simulink model "MRAC_111_8_5"  (Simulink 8.9)
settings: Solver=ode45  StartTime=0.0  StopTime=40.0  RelTol=1e-3  AbsTol=1e-6
values from neighbouring files (symbols this model uses):
  af = af2    [simu_gradiente.m]
  As = 0    [parameters.m]
  DC = 1    [parameters.m]
  gamma = gamma2    [simu_gradiente.m]
  m_type = 2    [simu_gradiente.m]
  st = 0.05    [simu_gradiente.m]
  theta0 = 0    [parameters.m]
  ws = 2    [parameters.m]
libraries: cstblocks x2
settings Model: Creator=Ramon  LastModifiedBy=renan
settings DataIOCC: LimitDataPoints=off  SaveOutput=off  SaveTime=off
settings OptimizationCC: BlockReduction=off  BooleanDataType=off  ExpressionDepthLimit=2147483647  InitFltsAndDblsToZero=on
settings DebuggingCC: SaveWithParameterizedLinksMsg=none  SignalResolutionControl=TryResolveAllWithWarning  MultiTaskDSMMsg=warning  MultiTaskCondExecSysMsg=none
settings HardwareCC: TargetUnknown=on
settings RTWCC: TemplateMakefile=grt_vc.tmf

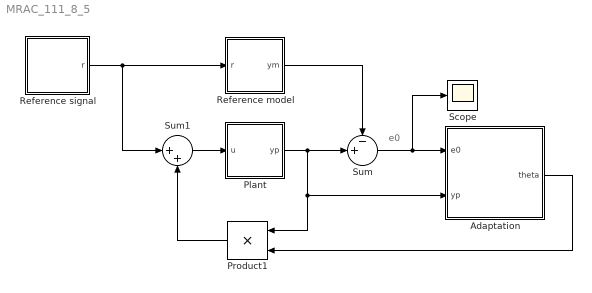
== system MRAC_111_8_5 ==
  note: e0
  Adaptation : Subsystem
  Plant : Subsystem
  Product1 : Product  SaturateOnIntegerOverflow=on  RndMeth=Zero  InputSameDT=on  OutDataTypeStr=Inherit: Same as first input
  Reference model : Subsystem
  Reference signal : Subsystem
  Scope : Scope
  Sum : Sum  Inputs=-+|  SaturateOnIntegerOverflow=on  InputSameDT=on  OutDataTypeStr=Inherit: Same as first input
  Sum1 : Sum  Inputs=|++  SaturateOnIntegerOverflow=on  InputSameDT=on  OutDataTypeStr=Inherit: Same as first input
  wires:
  Sum/1 -> Adaptation/1(e0), Scope/1
  Reference model/1(ym) -> Sum/1
  Plant/1(yp) -> Sum/2, Adaptation/2(yp), Product1/1
  Reference signal/1(r) -> Reference model/1(r), Sum1/1
  Sum1/1 -> Plant/1(u)
  Adaptation/1(theta) -> Product1/2
  Product1/1 -> Sum1/2

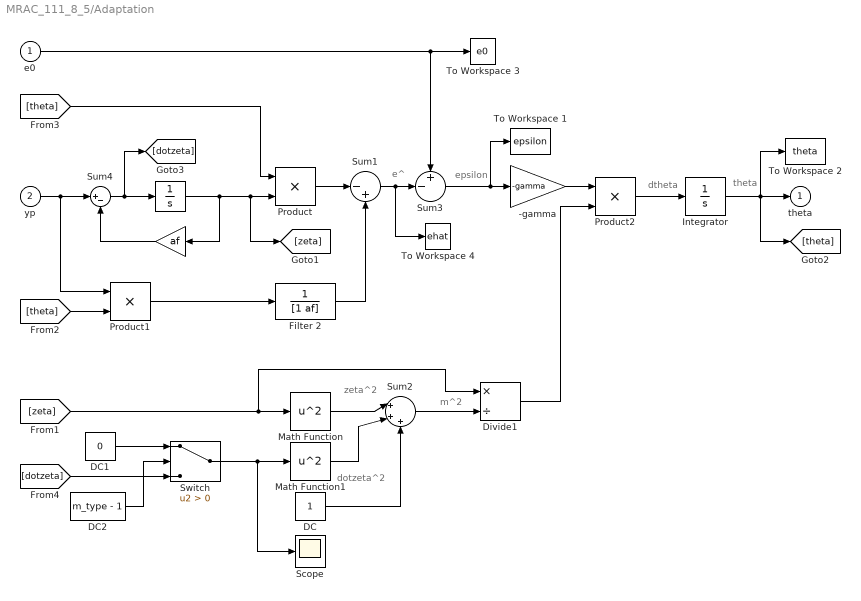
== system MRAC_111_8_5/Adaptation ==
  note: dotzeta^2
  note: theta
  note: dtheta
  note: epsilon
  note: zeta^2
  note: m^2
  note: e^
  e0 : Inport  PortDimensions=1
  yp : Inport  Port=2
  " " : Integrator
  "  " : Gain  Gain=af
  -gamma : Gain  Gain=-gamma  SaturateOnIntegerOverflow=on  OutDataTypeStr=Inherit: Same as input  ParamDataTypeStr=Inherit: Same as input
  DC : Constant
  DC1 : Constant  Value=0
  DC2 : Constant  Value=m_type - 1
  Divide1 : Product  Inputs=*/
  Filter 2 : TransferFcn  Denominator=[1 af]
  Integrator : Integrator  InitialCondition=theta0
  Math Function : Math  Operator=square  SaturateOnIntegerOverflow=on
  Math Function1 : Math  Operator=square  SaturateOnIntegerOverflow=on
  Product : Product  SaturateOnIntegerOverflow=on  RndMeth=Zero  InputSameDT=on  OutDataTypeStr=Inherit: Same as first input
  Product1 : Product  SaturateOnIntegerOverflow=on  RndMeth=Zero  InputSameDT=on  OutDataTypeStr=Inherit: Same as first input
  Product2 : Product  SaturateOnIntegerOverflow=on  RndMeth=Zero  InputSameDT=on  OutDataTypeStr=Inherit: Same as first input
  Scope : Scope
  Sum1 : Sum  Inputs=|-+  SaturateOnIntegerOverflow=on  InputSameDT=on  OutDataTypeStr=Inherit: Same as first input
  Sum2 : Sum  Inputs=|+++  SaturateOnIntegerOverflow=on  InputSameDT=on  OutDataTypeStr=Inherit: Same as first input
  Sum3 : Sum  Inputs=+-|  SaturateOnIntegerOverflow=on  InputSameDT=on  OutDataTypeStr=Inherit: Same as first input
  Sum4 : Sum  Inputs=|+-  SaturateOnIntegerOverflow=on  InputSameDT=on  OutDataTypeStr=Inherit: Same as first input
  Switch : Switch  Criteria=u2 > Threshold
  To Workspace 1 : ToWorkspace  VariableName=epsilon  SampleTime=st
  To Workspace 2 : ToWorkspace  VariableName=theta  SampleTime=st
  To Workspace 3 : ToWorkspace  VariableName=e0  SampleTime=st
  To Workspace 4 : ToWorkspace  VariableName=ehat  SampleTime=st
  theta : Outport  InitialOutput=0
  wires:
  yp/1 -> Sum4/1, Product1/1
  Product/1 -> Sum1/1
  Product1/1 -> Filter 2/1
  Filter 2/1 -> Sum1/2
  " "/1 -> "  "/1, [zeta], Product/2
  -gamma/1 -> Product2/1
  [zeta] -> Math Function/1, Divide1/1
  Sum2/1 -> Divide1/2
  Divide1/1 -> Product2/2
  Product2/1 -> Integrator/1
  Integrator/1 -> theta/1, To Workspace 2/1, [theta]
  e0/1 -> Sum3/1, To Workspace 3/1
  Sum1/1 -> Sum3/2, To Workspace 4/1
  Sum3/1 -> -gamma/1, To Workspace 1/1
  [theta] -> Product1/2
  [theta] -> Product/1
  Math Function/1 -> Sum2/1
  Sum4/1 -> " "/1, [dotzeta]
  "  "/1 -> Sum4/2
  DC/1 -> Sum2/3
  Math Function1/1 -> Sum2/2
  Switch/1 -> Scope/1, Math Function1/1
  DC2/1 -> Switch/2
  [dotzeta] -> Switch/3
  DC1/1 -> Switch/1

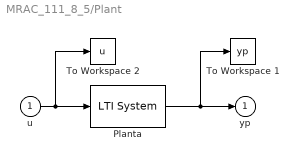
== system MRAC_111_8_5/Plant ==
  u : Inport
  Planta : cstblocks/LTI System  sys=P  IC=yp0
  To Workspace 1 : ToWorkspace  VariableName=yp  SampleTime=st
  To Workspace 2 : ToWorkspace  VariableName=u  SampleTime=st
  yp : Outport  InitialOutput=0
  wires:
  u/1 -> To Workspace 2/1, Planta/1
  Planta/1 -> yp/1, To Workspace 1/1

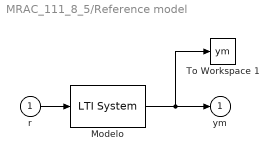
== system MRAC_111_8_5/Reference model ==
  r : Inport
  Modelo : cstblocks/LTI System  sys=M  IC=ym0
  To Workspace 1 : ToWorkspace  VariableName=ym  SampleTime=st
  ym : Outport  InitialOutput=0
  wires:
  Modelo/1 -> To Workspace 1/1, ym/1
  r/1 -> Modelo/1

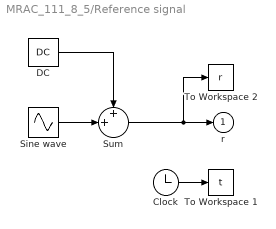
== system MRAC_111_8_5/Reference signal ==
  Clock : Clock
  DC : Constant  Value=DC
  Sine wave : Sin  Amplitude=As  Frequency=ws  SampleTime=0
  Sum : Sum  Inputs=++|  SaturateOnIntegerOverflow=on  InputSameDT=on  OutDataTypeStr=Inherit: Same as first input
  To Workspace 1 : ToWorkspace  VariableName=t  SampleTime=st
  To Workspace 2 : ToWorkspace  VariableName=r  SampleTime=st
  r : Outport  InitialOutput=0
  wires:
  DC/1 -> Sum/1
  Sum/1 -> r/1, To Workspace 2/1
  Clock/1 -> To Workspace 1/1
  Sine wave/1 -> Sum/2
